simulink model "n3_LTI_controller"  (R2023b)
settings: Solver=VariableStepAuto  StartTime=0.0  StopTime=80  RelTol=1e-3
values from neighbouring files (symbols this model uses):
  Alin = [0    -k/Jl + m*g*l*sin(x2_bar)/Jl                     0           k/Jl ... (first row only)    [collaborative_class_main.m]    (also in n0_collaborative_class_main.m = [ 0           -k/Jl + m*g*l*sin(x2_bar)/Jl             0    )
  Blin = [0; 0; 1/Jm; 0]    [collaborative_class_main.m]    (also in n0_collaborative_class_main.m)
  dx_0 = [0;1;0;1]*0.01    [n0_collaborative_class_main.m]    (also in svc_robot.m = [0;1;0;1]*0.1)
  K = place(Alin, Blin, p)    [collaborative_class_main.m]    (also in n0_collaborative_class_main.m)
  K_H2_V = K_H2(:, 5)    [collaborative_class_main.m]    (also in n0_collaborative_class_main.m)
  K_H2_X = K_H2(:,1:4)    [collaborative_class_main.m]    (also in n0_collaborative_class_main.m)
  K_lq = R^(-1)*Blin'*P_lq    [n0_collaborative_class_main.m]
  K_lqeta = K_lqe(:, 5)    [collaborative_class_main.m]    (also in n0_collaborative_class_main.m = K_lq_ext(:,5))
  K_lqx = K_lqe(:,1:4)    [collaborative_class_main.m]    (also in n0_collaborative_class_main.m = K_lq_ext(:,1:4))
  Kv = -K_ext(1, 5)    [collaborative_class_main.m]    (also in n0_collaborative_class_main.m)
  Kx = -K_ext(1, 1:4)    [collaborative_class_main.m]    (also in n0_collaborative_class_main.m)
  u_bar = m*g*l*cos(x2_bar)    [collaborative_class_main.m]    (also in n0_collaborative_class_main.m; svc_robot.m)
settings Model: Creator=teoma  LastModifiedBy=teoma

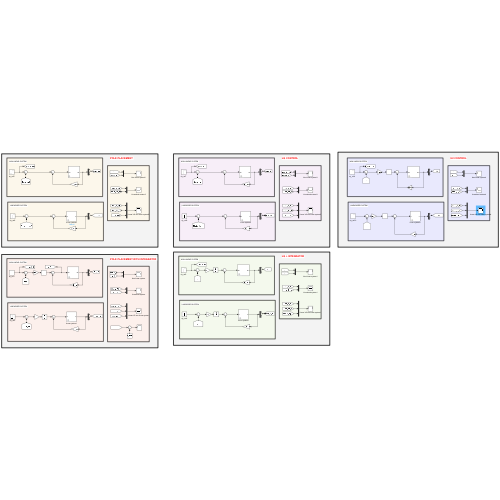
[thumbnail: Simulink's stored preview of the top-level diagram]
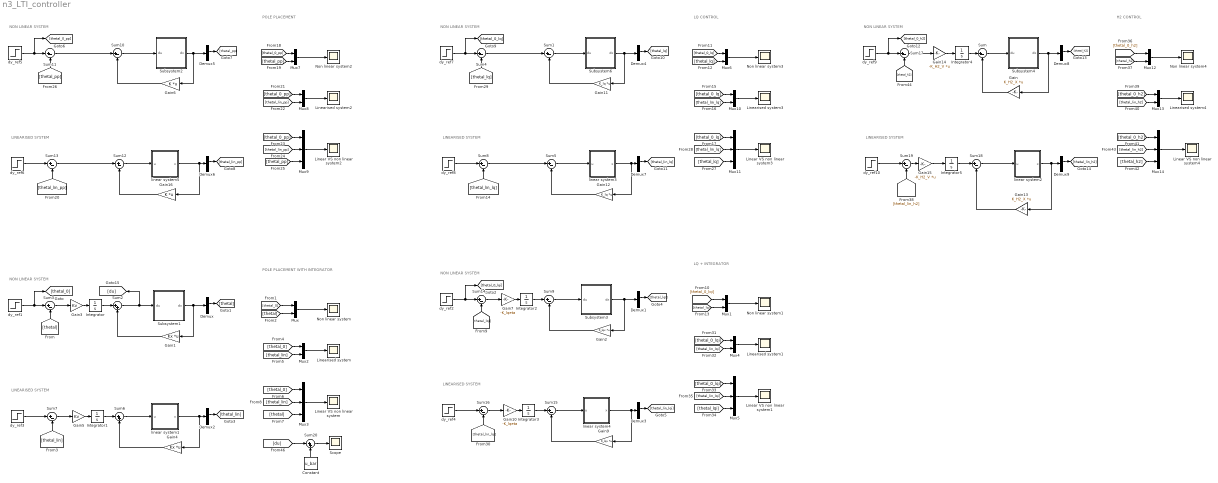
== system n3_LTI_controller ==
  note: LINEARISED SYSTEM
  note: LQ CONTROL
  note: LINEARISED SYSTEM
  note: NON LINEAR SYSTEM
  note: POLE PLACEMENT
  note: NON LINEAR SYSTEM
  note: LQ + INTEGRATOR
  note: LINEARISED SYSTEM
  note: POLE PLACEMENT WITH INTEGRATOR
  note: NON LINEAR SYSTEM
  note: LINEARISED SYSTEM
  note: NON LINEAR SYSTEM
  note: NON LINEAR SYSTEM
  note: H2 CONTROL
  note: LINEARISED SYSTEM
  Constant : Constant  Value=u_bar
  Demux{,1..9} (10 alike) : Demux
  Gain : Gain  Gain=K_H2_X  Multiplication=Matrix(K*u) (u vector)
  Gain1 : Gain  Gain=Kx  Multiplication=Matrix(K*u) (u vector)
  Gain10 : Gain  Gain=-K_lqeta
  Gain11 : Gain  Gain=K_lq  Multiplication=Matrix(K*u) (u vector)
  Gain12 : Gain  Gain=K_lq  Multiplication=Matrix(K*u) (u vector)
  Gain13 : Gain  Gain=K_H2_X  Multiplication=Matrix(K*u) (u vector)
  Gain14 : Gain  Gain=-K_H2_V  Multiplication=Matrix(K*u) (u vector)
  Gain15 : Gain  Gain=-K_H2_V  Multiplication=Matrix(K*u) (u vector)
  Gain16 : Gain  Gain=K  Multiplication=Matrix(K*u) (u vector)
  Gain2 : Gain  Gain=K_lqx  Multiplication=Matrix(K*u) (u vector)
  Gain3 : Gain  Gain=Kv
  Gain4 : Gain  Gain=Kx  Multiplication=Matrix(K*u) (u vector)
  Gain5 : Gain  Gain=Kv
  Gain6 : Gain  Gain=K  Multiplication=Matrix(K*u) (u vector)
  Gain7 : Gain  Gain=-K_lqeta
  Gain9 : Gain  Gain=K_lqx  Multiplication=Matrix(K*u) (u vector)
  Integrator{,1..5} (6 alike) : Integrator
  Linear VS non linear system{,1..4} (5 alike) : Scope
  Linearised system{,1..4} (5 alike) : Scope
  Mux{,1..2,4,6..8,10,12..13} (10 alike) : Mux  Inputs=2
  Mux{3,5,9,11,14} (5 alike) : Mux  Inputs=3
  Non linear system{,1..4} (5 alike) : Scope
  Scope : Scope
  Subsystem1 : Subsystem  mask{dx_0=dx_0}
      mask prompts: dx_0 "initial state"
  Subsystem2 : Subsystem  mask{dx_0=dx_0}
      mask prompts: dx_0 "initial state"
  Subsystem3 : Subsystem  mask{dx_0=dx_0}
      mask prompts: dx_0 "initial state"
  Subsystem4 : Subsystem  mask{dx_0=dx_0}
      mask prompts: dx_0 "initial state"
  Subsystem6 : Subsystem  mask{dx_0=dx_0}
      mask prompts: dx_0 "initial state"
  Sum{,1,3..5,7..19} (18 alike) : Sum  Inputs=|+-
  Sum2 : Sum  Inputs=|++
  Sum20 : Sum  Inputs=|++
  Sum6 : Sum  Inputs=|++
  dy_ref{1,3,5..6,9..10} (6 alike) : Step  After=pi/36  SampleTime=0
  dy_ref{2,4,7..8} (4 alike) : Step  Time=0  After=pi/36  SampleTime=0
  linear system1 : Subsystem  mask{dx_0=dx_0}
      mask prompts: dx_0 "initial state"
  linear system2 : Subsystem  mask{dx_0=dx_0}
      mask prompts: dx_0 "initial state"
  linear system3 : Subsystem  mask{dx_0=dx_0}
      mask prompts: dx_0 "initial state"
  linear system4 : Subsystem  mask{dx_0=dx_0}
      mask prompts: dx_0 "initial state"
  linear system5 : Subsystem  mask{dx_0=dx_0}
      mask prompts: dx_0 "initial state"
  wires:
  [thetal_0_pp] -> Mux8/1
  [thetal_lin_h2] -> Mux14/2
  Gain15/1 -> Integrator5/1
  [thetal_0_lqi] -> Mux5/1
  [thetal_0_h2] -> Mux13/1
  dy_ref2/1 -> [thetal_0_lqi], Sum14/1
  Mux2/1 -> Linearised system/1
  Mux4/1 -> Linearised system1/1
  [thetal_h2] -> Mux14/3
  dy_ref9/1 -> [thetal_0_h2], Sum17/1
  Integrator4/1 -> Sum/1
  Sum20/1 -> Scope/1
  Mux6/1 -> Non linear system3/1
  [thetal_lin_h2] -> Mux13/2
  Sum19/1 -> Gain15/1
  [thetal_lin_lqi] -> Mux4/2
  Gain/1 -> Sum/2
  Integrator5/1 -> Sum18/1
  Mux7/1 -> Non linear system2/1
  Sum9/1 -> Subsystem3/1(du)
  [thetal_lq] -> Mux6/2
  linear system3/1(x) -> Gain12/1, Demux7/1
  Sum18/1 -> linear system2/1(u)
  Sum17/1 -> Gain14/1
  Gain2/1 -> Sum9/2
  Mux13/1 -> Linearised system4/1
  Subsystem6/1(dx) -> Gain11/1, Demux4/1
  [thetal_lin_lq] -> Mux10/2
  Demux7/2 -> [thetal_lin_lq]
  [thetal_h2] -> Mux12/2
  linear system2/1(x) -> Gain13/1, Demux9/1
  Sum7/1 -> Gain5/1
  Gain11/1 -> Sum1/2
  [thetal_lin_h2] -> Sum19/2
  Gain13/1 -> Sum18/2
  Demux4/2 -> [thetal_lq]
  Mux14/1 -> Linear VS non linear system4/1
  dy_ref4/1 -> Sum16/1
  [thetal_0_h2] -> Mux12/1
  Gain10/1 -> Integrator3/1
  Demux9/2 -> [thetal_lin_h2]
  Mux8/1 -> Linearised system2/1
  dy_ref3/1 -> Sum7/1
  [thetal_h2] -> Sum17/2
  Mux12/1 -> Non linear system4/1
  Sum1/1 -> Subsystem6/1(du)
  [thetal_0] -> Mux3/1
  dy_ref7/1 -> [thetal_0_lq], Sum4/1
  [thetal_lin_lqi] -> Sum16/2
  Gain12/1 -> Sum5/2
  [thetal_lqi] -> Mux5/3
  Sum15/1 -> linear system4/1(u)
  [thetal_0_h2] -> Mux14/1
  Sum4/1 -> Sum1/1
  Demux8/2 -> [thetal_h2]
  dy_ref10/1 -> Sum19/1
  Integrator2/1 -> Sum9/1
  Mux5/1 -> Linear VS non linear system1/1
  [thetal_lin_lq] -> Mux11/2
  Mux11/1 -> Linear VS non linear system3/1
  Sum12/1 -> linear system5/1(u)
  Mux3/1 -> Linear VS non linear system/1
  Sum14/1 -> Gain7/1
  [thetal_0_lq] -> Mux11/1
  Subsystem3/1(dx) -> Gain2/1, Demux1/1
  dy_ref8/1 -> Sum8/1
  [thetal_lqi] -> Sum14/2
  Gain4/1 -> Sum6/2
  Demux5/2 -> [thetal_pp]
  [thetal_lq] -> Sum4/2
  [thetal_lqi] -> Mux1/2
  Demux2/2 -> [thetal_lin]
  Subsystem4/1(dx) -> Gain/1, Demux8/1
  [thetal] -> Mux/2
  linear system4/1(x) -> Gain9/1, Demux3/1
  Sum16/1 -> Gain10/1
  Gain9/1 -> Sum15/2
  Demux/2 -> [thetal]
  Sum5/1 -> linear system3/1(u)
  [thetal] -> Mux3/3
  Sum3/1 -> Gain3/1
  Gain7/1 -> Integrator2/1
  Gain14/1 -> Integrator4/1
  Gain6/1 -> Sum10/2
  [thetal_lin] -> Sum7/2
  [thetal_0_lqi] -> Mux4/1
  [thetal_pp] -> Sum11/2
  [thetal_0_lq] -> Mux10/1
  Sum6/1 -> linear system1/1(u)
  Gain5/1 -> Integrator1/1
  [du] -> Sum20/1
  Demux1/2 -> [thetal_lqi]
  [thetal_0_lq] -> Mux6/1
  [thetal_lin_pp] -> Mux9/2
  Sum13/1 -> Sum12/1
  Mux1/1 -> Non linear system1/1
  Sum/1 -> Subsystem4/1(du)
  [thetal_lq] -> Mux11/3
  Sum11/1 -> Sum10/1
  Mux10/1 -> Linearised system3/1
  Demux3/2 -> [thetal_lin_lqi]
  [thetal_pp] -> Mux9/3
  Integrator3/1 -> Sum15/1
  Demux6/2 -> [thetal_lin_pp]
  [thetal_lin_pp] -> Sum13/2
  [thetal_0_pp] -> Mux7/1
  Sum8/1 -> Sum5/1
  Mux9/1 -> Linear VS non linear system2/1
  Gain16/1 -> Sum12/2
  dy_ref1/1 -> [thetal_0], Sum3/1
  linear system5/1(x) -> Gain16/1, Demux6/1
  dy_ref5/1 -> [thetal_0_pp], Sum11/1
  Constant/1 -> Sum20/2
  [thetal_lin_pp] -> Mux8/2
  [thetal_pp] -> Mux7/2
  [thetal_0_pp] -> Mux9/1
  Subsystem2/1(dx) -> Gain6/1, Demux5/1
  [thetal_lin] -> Mux3/2
  Integrator1/1 -> Sum6/1
  Sum10/1 -> Subsystem2/1(du)
  [thetal_0] -> Mux2/1
  linear system1/1(x) -> Gain4/1, Demux2/1
  Integrator/1 -> Sum2/1
  Gain3/1 -> Integrator/1
  [thetal_lin] -> Mux2/2
  [thetal_lin_lq] -> Sum8/2
  Subsystem1/1(dx) -> Gain1/1, Demux/1
  [thetal] -> Sum3/2
  [thetal_0_lqi] -> Mux1/1
  [thetal_0] -> Mux/1
  Sum2/1 -> [du], Subsystem1/1(du)
  [thetal_lin_lqi] -> Mux5/2
  Mux/1 -> Non linear system/1
  Gain1/1 -> Sum2/2
  dy_ref6/1 -> Sum13/1

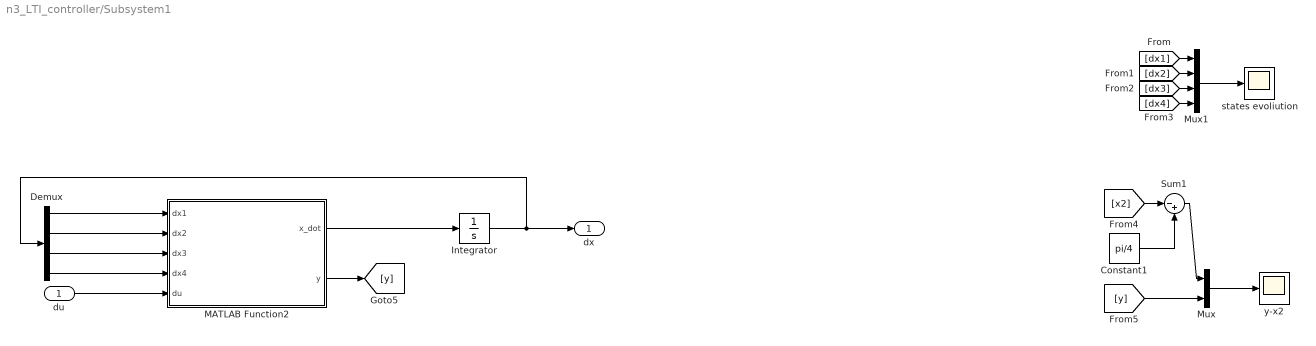
== system n3_LTI_controller/Subsystem1 ==
  du : Inport
  Constant1 : Constant  Value=pi/4
  Demux : Demux
  Integrator : Integrator  InitialCondition=dx_0
  MATLAB Function2 : MATLAB Function  TreatAsAtomicUnit=on
  Mux : Mux  Inputs=2
  Mux1 : Mux
  Sum1 : Sum  Inputs=|-+
  "states evoliution " : Scope
  y-x2 : Scope
  dx : Outport
  wires:
  du/1 -> MATLAB Function2/5(du)
  MATLAB Function2/2(y) -> [y]
  Demux/1 -> MATLAB Function2/1(dx1)
  Demux/2 -> MATLAB Function2/2(dx2)
  Demux/3 -> MATLAB Function2/3(dx3)
  Demux/4 -> MATLAB Function2/4(dx4)
  MATLAB Function2/1(x_dot) -> Integrator/1
  Integrator/1 -> dx/1, Demux/1
  Mux/1 -> y-x2/1
  Sum1/1 -> Mux/1
  Constant1/1 -> Sum1/2
  [dx1] -> Mux1/1
  [dx2] -> Mux1/2
  [dx3] -> Mux1/3
  [dx4] -> Mux1/4
  Mux1/1 -> "states evoliution "/1
  [x2] -> Sum1/1
  [y] -> Mux/2

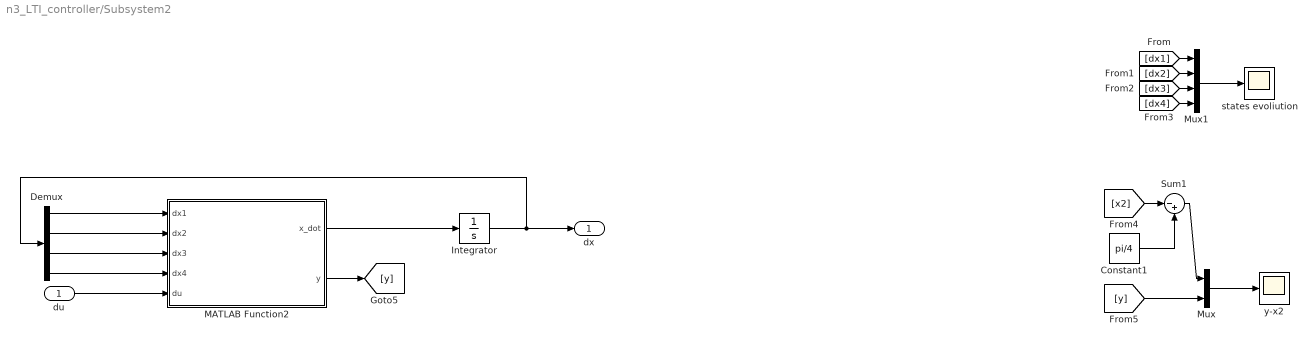
== system n3_LTI_controller/Subsystem2 ==
  du : Inport
  Constant1 : Constant  Value=pi/4
  Demux : Demux
  Integrator : Integrator  InitialCondition=dx_0
  MATLAB Function2 : MATLAB Function  TreatAsAtomicUnit=on
  Mux : Mux  Inputs=2
  Mux1 : Mux
  Sum1 : Sum  Inputs=|-+
  "states evoliution " : Scope
  y-x2 : Scope
  dx : Outport
  wires:
  du/1 -> MATLAB Function2/5(du)
  MATLAB Function2/2(y) -> [y]
  Demux/1 -> MATLAB Function2/1(dx1)
  Demux/2 -> MATLAB Function2/2(dx2)
  Demux/3 -> MATLAB Function2/3(dx3)
  Demux/4 -> MATLAB Function2/4(dx4)
  MATLAB Function2/1(x_dot) -> Integrator/1
  Integrator/1 -> dx/1, Demux/1
  Mux/1 -> y-x2/1
  Sum1/1 -> Mux/1
  Constant1/1 -> Sum1/2
  [dx1] -> Mux1/1
  [dx2] -> Mux1/2
  [dx3] -> Mux1/3
  [dx4] -> Mux1/4
  Mux1/1 -> "states evoliution "/1
  [x2] -> Sum1/1
  [y] -> Mux/2

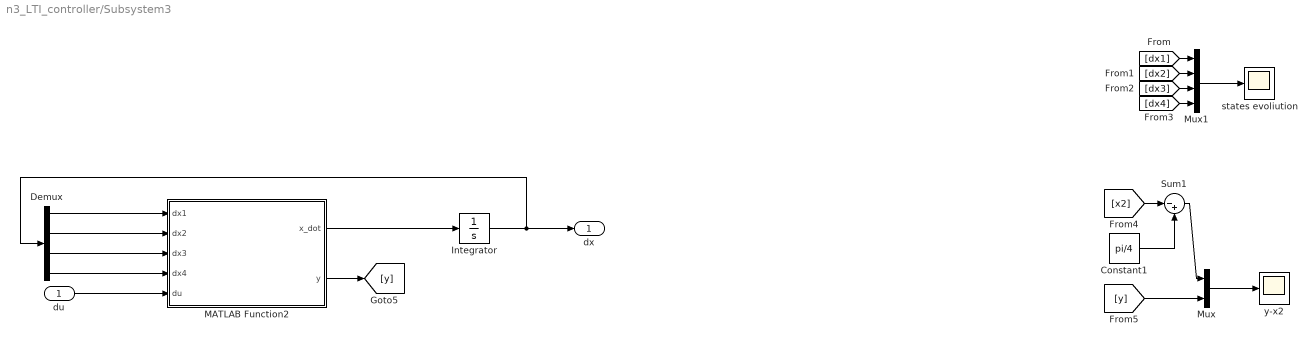
== system n3_LTI_controller/Subsystem3 ==
  du : Inport
  Constant1 : Constant  Value=pi/4
  Demux : Demux
  Integrator : Integrator  InitialCondition=dx_0
  MATLAB Function2 : MATLAB Function  TreatAsAtomicUnit=on
  Mux : Mux  Inputs=2
  Mux1 : Mux
  Sum1 : Sum  Inputs=|-+
  "states evoliution " : Scope
  y-x2 : Scope
  dx : Outport
  wires:
  du/1 -> MATLAB Function2/5(du)
  MATLAB Function2/2(y) -> [y]
  Demux/1 -> MATLAB Function2/1(dx1)
  Demux/2 -> MATLAB Function2/2(dx2)
  Demux/3 -> MATLAB Function2/3(dx3)
  Demux/4 -> MATLAB Function2/4(dx4)
  MATLAB Function2/1(x_dot) -> Integrator/1
  Integrator/1 -> dx/1, Demux/1
  Mux/1 -> y-x2/1
  Sum1/1 -> Mux/1
  Constant1/1 -> Sum1/2
  [dx1] -> Mux1/1
  [dx2] -> Mux1/2
  [dx3] -> Mux1/3
  [dx4] -> Mux1/4
  Mux1/1 -> "states evoliution "/1
  [x2] -> Sum1/1
  [y] -> Mux/2

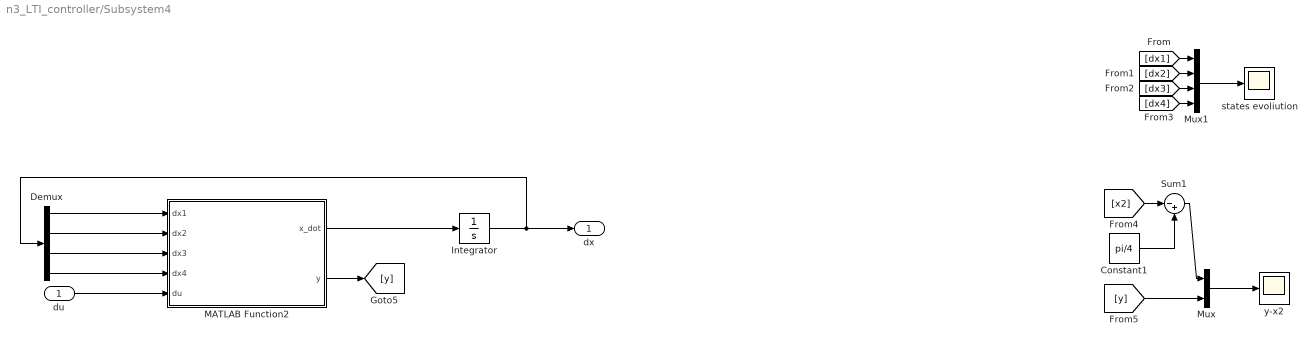
== system n3_LTI_controller/Subsystem4 ==
  du : Inport
  Constant1 : Constant  Value=pi/4
  Demux : Demux
  Integrator : Integrator  InitialCondition=dx_0
  MATLAB Function2 : MATLAB Function  TreatAsAtomicUnit=on
  Mux : Mux  Inputs=2
  Mux1 : Mux
  Sum1 : Sum  Inputs=|-+
  "states evoliution " : Scope
  y-x2 : Scope
  dx : Outport
  wires:
  du/1 -> MATLAB Function2/5(du)
  MATLAB Function2/2(y) -> [y]
  Demux/1 -> MATLAB Function2/1(dx1)
  Demux/2 -> MATLAB Function2/2(dx2)
  Demux/3 -> MATLAB Function2/3(dx3)
  Demux/4 -> MATLAB Function2/4(dx4)
  MATLAB Function2/1(x_dot) -> Integrator/1
  Integrator/1 -> dx/1, Demux/1
  Mux/1 -> y-x2/1
  Sum1/1 -> Mux/1
  Constant1/1 -> Sum1/2
  [dx1] -> Mux1/1
  [dx2] -> Mux1/2
  [dx3] -> Mux1/3
  [dx4] -> Mux1/4
  Mux1/1 -> "states evoliution "/1
  [x2] -> Sum1/1
  [y] -> Mux/2

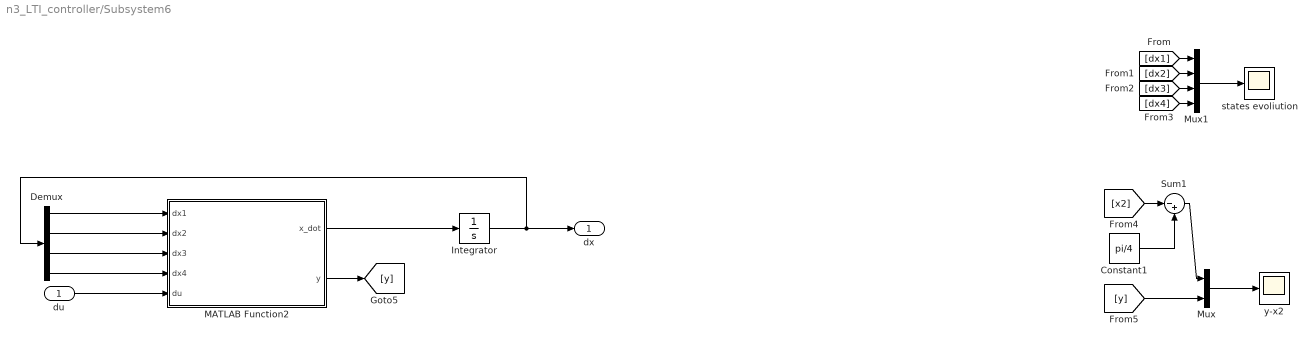
== system n3_LTI_controller/Subsystem6 ==
  du : Inport
  Constant1 : Constant  Value=pi/4
  Demux : Demux
  Integrator : Integrator  InitialCondition=dx_0
  MATLAB Function2 : MATLAB Function  TreatAsAtomicUnit=on
  Mux : Mux  Inputs=2
  Mux1 : Mux
  Sum1 : Sum  Inputs=|-+
  "states evoliution " : Scope
  y-x2 : Scope
  dx : Outport
  wires:
  du/1 -> MATLAB Function2/5(du)
  MATLAB Function2/2(y) -> [y]
  Demux/1 -> MATLAB Function2/1(dx1)
  Demux/2 -> MATLAB Function2/2(dx2)
  Demux/3 -> MATLAB Function2/3(dx3)
  Demux/4 -> MATLAB Function2/4(dx4)
  MATLAB Function2/1(x_dot) -> Integrator/1
  Integrator/1 -> dx/1, Demux/1
  Mux/1 -> y-x2/1
  Sum1/1 -> Mux/1
  Constant1/1 -> Sum1/2
  [dx1] -> Mux1/1
  [dx2] -> Mux1/2
  [dx3] -> Mux1/3
  [dx4] -> Mux1/4
  Mux1/1 -> "states evoliution "/1
  [x2] -> Sum1/1
  [y] -> Mux/2

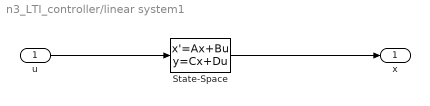
== system n3_LTI_controller/linear system1 ==
  u : Inport
  State-Space : StateSpace  A=Alin  B=Blin  C=eye(4)  D=zeros(4,1)  InitialCondition=dx_0
  x : Outport
  wires:
  State-Space/1 -> x/1
  u/1 -> State-Space/1

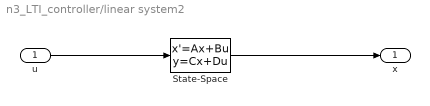
== system n3_LTI_controller/linear system2 ==
  u : Inport
  State-Space : StateSpace  A=Alin  B=Blin  C=eye(4)  D=zeros(4,1)  InitialCondition=dx_0
  x : Outport
  wires:
  State-Space/1 -> x/1
  u/1 -> State-Space/1

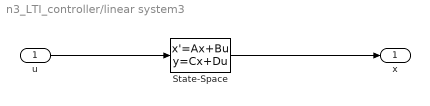
== system n3_LTI_controller/linear system3 ==
  u : Inport
  State-Space : StateSpace  A=Alin  B=Blin  C=eye(4)  D=zeros(4,1)  InitialCondition=dx_0
  x : Outport
  wires:
  State-Space/1 -> x/1
  u/1 -> State-Space/1

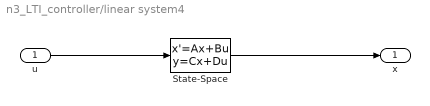
== system n3_LTI_controller/linear system4 ==
  u : Inport
  State-Space : StateSpace  A=Alin  B=Blin  C=eye(4)  D=zeros(4,1)  InitialCondition=dx_0
  x : Outport
  wires:
  State-Space/1 -> x/1
  u/1 -> State-Space/1

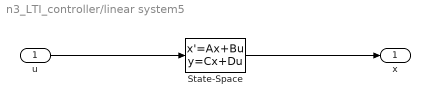
== system n3_LTI_controller/linear system5 ==
  u : Inport
  State-Space : StateSpace  A=Alin  B=Blin  C=eye(4)  D=zeros(4,1)  InitialCondition=dx_0
  x : Outport
  wires:
  State-Space/1 -> x/1
  u/1 -> State-Space/1

== matlab function n3_LTI_controller/Subsystem3/MATLAB Function2 ==
  data: dx1 input; dx2 input; dx3 input; dx4 input; du input; x_dot output; y output
function [x_dot, y]  = fcn(dx1,dx2,dx3,dx4, du)

k = 0.8;
Jm = 4e-4;
Jl= 4e-4;
Bm = 0.015;
Bl = 0;
m = 0.3;
l = 0.3;
g = 9.81;
x1_bar = 0;
x2_bar = pi/4;
x3_bar = 0;
x4_bar = m*g*l*cos(x2_bar)/k + x2_bar;
u_bar= m*g*l*cos(x2_bar);


x1_dot = -k/Jl*(dx2+x2_bar)-m*g*l/Jl*(cos(dx2+x2_bar))+k/Jl*(dx4+x4_bar);
x2_dot = dx1+x1_bar;
x3_dot = k/Jm*(dx2+x2_bar)-Bm/Jm*(dx3+x3_bar)-k/Jm*(dx4+x4_bar)+1/Jm*(du+u_bar);
x4_dot = dx3+x3_bar;
y = pi/4 - (dx2+x2_bar);

x_dot = zeros(1,4);
x_dot(1) = x1_dot;
x_dot(2) = x2_dot;
x_dot(3) = x3_dot;
x_dot(4) = x4_dot;

== matlab function n3_LTI_controller/Subsystem2/MATLAB Function2 ==
  data: dx1 input; dx2 input; dx3 input; dx4 input; du input; x_dot output; y output
function [x_dot, y]  = fcn(dx1,dx2,dx3,dx4, du)

k = 0.8;
Jm = 4e-4;
Jl= 4e-4;
Bm = 0.015;
Bl = 0;
m = 0.3;
l = 0.3;
g = 9.81;
x1_bar = 0;
x2_bar = pi/4;
x3_bar = 0;
x4_bar = m*g*l*cos(x2_bar)/k + x2_bar;
u_bar= m*g*l*cos(x2_bar);


x1_dot = -k/Jl*(dx2+x2_bar)-m*g*l/Jl*(cos(dx2+x2_bar))+k/Jl*(dx4+x4_bar);
x2_dot = dx1+x1_bar;
x3_dot = k/Jm*(dx2+x2_bar)-Bm/Jm*(dx3+x3_bar)-k/Jm*(dx4+x4_bar)+1/Jm*(du+u_bar);
x4_dot = dx3+x3_bar;
y = pi/4 - (dx2+x2_bar);

x_dot = zeros(1,4);
x_dot(1) = x1_dot;
x_dot(2) = x2_dot;
x_dot(3) = x3_dot;
x_dot(4) = x4_dot;

== matlab function n3_LTI_controller/Subsystem4/MATLAB Function2 ==
  data: dx1 input; dx2 input; dx3 input; dx4 input; du input; x_dot output; y output
function [x_dot, y]  = fcn(dx1,dx2,dx3,dx4, du)

k = 0.8;
Jm = 4e-4;
Jl= 4e-4;
Bm = 0.015;
Bl = 0;
m = 0.3;
l = 0.3;
g = 9.81;
x1_bar = 0;
x2_bar = pi/4;
x3_bar = 0;
x4_bar = m*g*l*cos(x2_bar)/k + x2_bar;
u_bar= m*g*l*cos(x2_bar);


x1_dot = -k/Jl*(dx2+x2_bar)-m*g*l/Jl*(cos(dx2+x2_bar))+k/Jl*(dx4+x4_bar);
x2_dot = dx1+x1_bar;
x3_dot = k/Jm*(dx2+x2_bar)-Bm/Jm*(dx3+x3_bar)-k/Jm*(dx4+x4_bar)+1/Jm*(du+u_bar);
x4_dot = dx3+x3_bar;
y = pi/4 - (dx2+x2_bar);

x_dot = zeros(1,4);
x_dot(1) = x1_dot;
x_dot(2) = x2_dot;
x_dot(3) = x3_dot;
x_dot(4) = x4_dot;

== matlab function n3_LTI_controller/Subsystem1/MATLAB Function2 ==
  data: dx1 input; dx2 input; dx3 input; dx4 input; du input; x_dot output; y output
function [x_dot, y]  = fcn(dx1,dx2,dx3,dx4, du)

k = 0.8;
Jm = 4e-4;
Jl= 4e-4;
Bm = 0.015;
Bl = 0;
m = 0.3;
l = 0.3;
g = 9.81;
x1_bar = 0;
x2_bar = pi/4;
x3_bar = 0;
x4_bar = m*g*l*cos(x2_bar)/k + x2_bar;
u_bar= m*g*l*cos(x2_bar);


x1_dot = -k/Jl*(dx2+x2_bar)-m*g*l/Jl*(cos(dx2+x2_bar))+k/Jl*(dx4+x4_bar);
x2_dot = dx1+x1_bar;
x3_dot = k/Jm*(dx2+x2_bar)-Bm/Jm*(dx3+x3_bar)-k/Jm*(dx4+x4_bar)+1/Jm*(du+u_bar);
x4_dot = dx3+x3_bar;
y = pi/4 - (dx2+x2_bar);

x_dot = zeros(1,4);
x_dot(1) = x1_dot;
x_dot(2) = x2_dot;
x_dot(3) = x3_dot;
x_dot(4) = x4_dot;

== matlab function n3_LTI_controller/Subsystem6/MATLAB Function2 ==
  data: dx1 input; dx2 input; dx3 input; dx4 input; du input; x_dot output; y output
function [x_dot, y]  = fcn(dx1,dx2,dx3,dx4, du)

k = 0.8;
Jm = 4e-4;
Jl= 4e-4;
Bm = 0.015;
Bl = 0;
m = 0.3;
l = 0.3;
g = 9.81;
x1_bar = 0;
x2_bar = pi/4;
x3_bar = 0;
x4_bar = m*g*l*cos(x2_bar)/k + x2_bar;
u_bar= m*g*l*cos(x2_bar);


x1_dot = -k/Jl*(dx2+x2_bar)-m*g*l/Jl*(cos(dx2+x2_bar))+k/Jl*(dx4+x4_bar);
x2_dot = dx1+x1_bar;
x3_dot = k/Jm*(dx2+x2_bar)-Bm/Jm*(dx3+x3_bar)-k/Jm*(dx4+x4_bar)+1/Jm*(du+u_bar);
x4_dot = dx3+x3_bar;
y = pi/4 - (dx2+x2_bar);

x_dot = zeros(1,4);
x_dot(1) = x1_dot;
x_dot(2) = x2_dot;
x_dot(3) = x3_dot;
x_dot(4) = x4_dot;
